simulink model "untitled"  (R2025b)
settings: Solver=VariableStepAuto  StartTime=0.0  StopTime=10.0  RelTol=1e-3
values from neighbouring files (symbols this model uses):
  K = [2.2360679775  -3.63559992725e-16  2.72862768324e-16; 1.21237084823e-16  4.08248290464  2.65354085926]    [thetad.mat]    (also in vd.mat; wd.mat; yd.mat)
  L = 0.4    [thetad.mat]    (also in vd.mat; wd.mat; yd.mat)
libraries: simulink x4, slpidlib x2
settings Model: Creator=mwali  LastModifiedBy=mwali

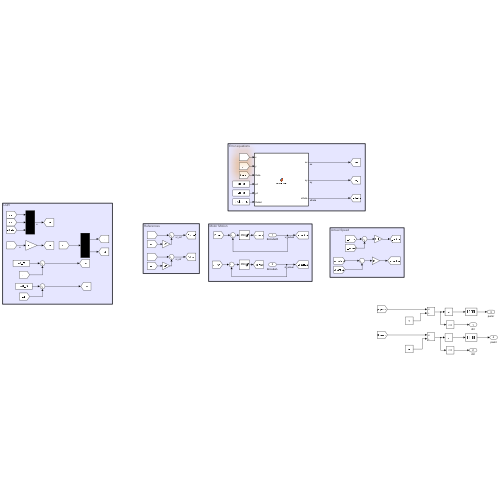
[thumbnail: Simulink's stored preview of the top-level diagram]
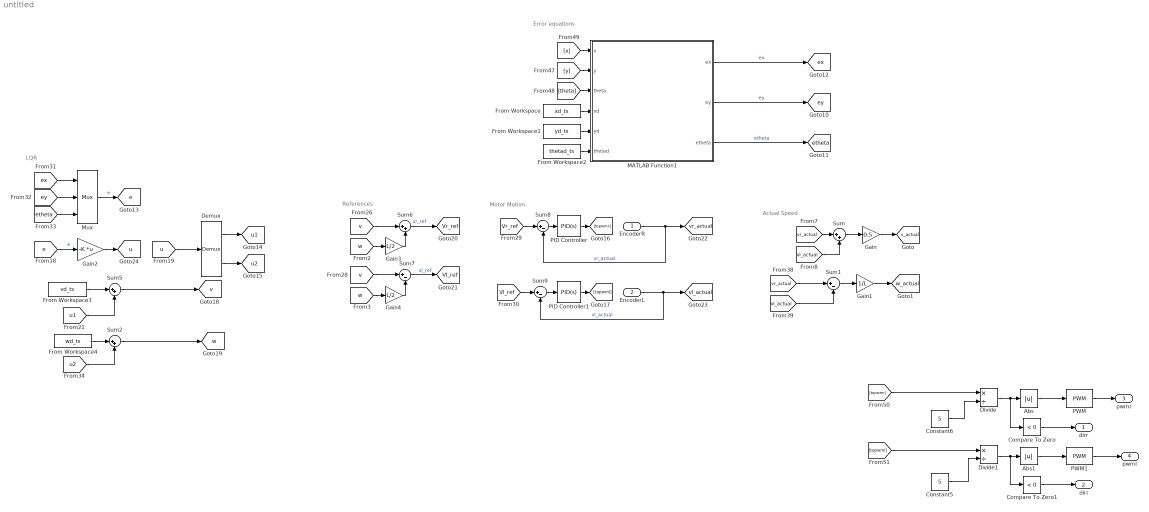
== system untitled ==
  note: LQR
  note: Actual Speed
  note: Error equations
  note: Motor Motion
  note: References
  EncoderR : Inport
  EncoderL : Inport  Port=2
  Abs : Abs  SaturateOnIntegerOverflow=off
  Abs1 : Abs  SaturateOnIntegerOverflow=off
  Compare To Zero : simulink/Logic and Bit Operations/Compare To Zero  relop=<  OutDataTypeStr=boolean
  Compare To Zero1 : simulink/Logic and Bit Operations/Compare To Zero  relop=<  OutDataTypeStr=boolean
  Constant5 : Constant  Value=5
  Constant6 : Constant  Value=5
  Demux : Demux  Outputs=2
  Divide : Product  Inputs=*/
  Divide1 : Product  Inputs=*/
  From Workspace : FromWorkspace  VariableName=xd_ts
  From Workspace1 : FromWorkspace  VariableName=yd_ts
  From Workspace2 : FromWorkspace  VariableName=thetad_ts
  From Workspace3 : FromWorkspace  VariableName=vd_ts
  From Workspace4 : FromWorkspace  VariableName=wd_ts
  Gain : Gain  Gain=0.5
  Gain1 : Gain  Gain=1/L
  Gain2 : Gain  Gain=-K  Multiplication=Matrix(K*u)
  Gain3 : Gain  Gain=L/2
  Gain4 : Gain  Gain=L/2
  MATLAB Function1 : MATLAB Function  TreatAsAtomicUnit=on
  Mux : Mux  Inputs=3
  PID Controller : slpidlib/PID Controller  Controller=PID  Form=Parallel  TimeDomain=Continuous-time  UseExternalTs=off  SampleTime=-1  IntegratorMethod=Forward Euler  FilterMethod=Forward Euler  ControllerParametersSource=internal  P=5  I=0.07  UseKiTs=off  D=0  UseExternalDerivativeSource=off  N=100  UseFilter=on  TunerSelectOption=Transfer Function Based (PID Tuner App)  InitialConditionSource=internal  InitialConditionForIntegrator=0  InitialConditionForFilter=0  DifferentiatorICPrevScaledInput=0  ExternalReset=none  TrackingMode=off  Kt=1  LimitOutput=on  SatLimitsSource=internal  UpperSaturationLimit=5  LowerSaturationLimit=-5  LinearizeAsGain=on  AntiWindupMode=clamping  Kb=1  LimitIntegrator=off  UpperIntegratorSaturationLimit=inf  LowerIntegratorSaturationLimit=-inf  POutMin=[]  POutMax=[]  IOutMin=[]  IOutMax=[]  DOutMin=[]  DOutMax=[]  NOutMin=[]  NOutMax=[]  SumOutMin=[]  SumOutMax=[]  SaturationOutMin=[]  SaturationOutMax=[]  PParamMin=[]  PParamMax=[]  IParamMin=[]  IParamMax=[]  DParamMin=[]  DParamMax=[]  NParamMin=[]  NParamMax=[]  KbParamMin=[]  KbParamMax=[]  KtParamMin=[]  KtParamMax=[]  KbOutMin=[]  KbOutMax=[]  KtOutMin=[]  KtOutMax=[]  IntegratorOutMin=[]  IntegratorOutMax=[]  FilterOutMin=[]  FilterOutMax=[]  SumI1OutMin=[]  SumI1OutMax=[]  SumI2OutMin=[]  SumI2OutMax=[]  SumI3OutMin=[]  SumI3OutMax=[]  SumI4OutMin=[]  SumI4OutMax=[]  SumDOutMin=[]  SumDOutMax=[]  DifferentiatorOutMin=[]  DifferentiatorOutMax=[]  FilterDiffOutCoefMin=[]  FilterDiffOutCoefMax=[]  ReciprocalOutMin=[]  ReciprocalOutMax=[]  SumDenOutMin=[]  SumDenOutMax=[]  SumNumOutMin=[]  SumNumOutMax=[]  DivideOutMin=[]  DivideOutMax=[]  UdiffTsProdOutMin=[]  UdiffTsProdOutMax=[]  NTsProdOutMin=[]  NTsProdOutMax=[]  UintegralTsProdOutMin=[]  UintegralTsProdOutMax=[]  UngainTsProdOutMin=[]  UngainTsProdOutMax=[]  ClampingZeroOutDataTypeStr=Inherit: Inherit via back propagation  ClampingZeroOutMin=[]  ClampingZeroOutMax=[]  FilterDenConstantOutDataTypeStr=Inherit: Inherit via back propagation  FilterDenConstantOutMin=[]  FilterDenConstantOutMax=[]  PCopyOutDataTypeStr=Inherit: Inherit via back propagation  PCopyOutMin=[]  PCopyOutMax=[]  NCopyOutDataTypeStr=Inherit: Inherit via back propagation  NCopyOutMin=[]  NCopyOutMax=[]  IntegratorContinuousStateAttributes=''  IntegratorStateMustResolveToSignalObject=off  IntegratorRTWStateStorageClass=Auto  FilterContinuousStateAttributes=''  FilterStateMustResolveToSignalObject=off  FilterRTWStateStorageClass=Auto  ParallelPVariant=InternalParameters  IdealPVariant=Disabled  IVariant=InternalParameters  DVariant=InternalParameters  IntegratorVariant=Continuous  SatVariant=Enabled  AWVariant=ContClampingParallel  PCopyVariant=Disabled  TRVariant=Disabled  FdbkBlocksVariant=Forward  IdealPFdbkVariant=Disabled  SatFdbkVariant=Disabled  DerivativeFilterVariant=ContFilter  NVariant=InternalParameters  NCopyVariant=Disabled  FilterICVariant=InternalICsFilter  IntegratorICVariant=InternalICs  ExternalResetVariant=Disabled  TRSumVariant=Passthrough  SumFdbkVariant=Disabled  SumVariant=Sum_PID  TsampFilterVariant=InternalTs  TsampNgainVariant=Passthrough  TsampIntegralVariant=Disabled_SignalSpec  ExternalSaturationOutDataTypeStr=Inherit: Same as second input  DerivativeSourceVariant=ErrorSignal  PreIntVariant=InternalPreInt
  PID Controller1 : slpidlib/PID Controller  Controller=PID  Form=Parallel  TimeDomain=Continuous-time  UseExternalTs=off  SampleTime=-1  IntegratorMethod=Forward Euler  FilterMethod=Forward Euler  ControllerParametersSource=internal  P=5  I=0.07  UseKiTs=off  D=0  UseExternalDerivativeSource=off  N=100  UseFilter=on  TunerSelectOption=Transfer Function Based (PID Tuner App)  InitialConditionSource=internal  InitialConditionForIntegrator=0  InitialConditionForFilter=0  DifferentiatorICPrevScaledInput=0  ExternalReset=none  TrackingMode=off  Kt=1  LimitOutput=on  SatLimitsSource=internal  UpperSaturationLimit=5  LowerSaturationLimit=-5  LinearizeAsGain=on  AntiWindupMode=clamping  Kb=1  LimitIntegrator=off  UpperIntegratorSaturationLimit=inf  LowerIntegratorSaturationLimit=-inf  POutMin=[]  POutMax=[]  IOutMin=[]  IOutMax=[]  DOutMin=[]  DOutMax=[]  NOutMin=[]  NOutMax=[]  SumOutMin=[]  SumOutMax=[]  SaturationOutMin=[]  SaturationOutMax=[]  PParamMin=[]  PParamMax=[]  IParamMin=[]  IParamMax=[]  DParamMin=[]  DParamMax=[]  NParamMin=[]  NParamMax=[]  KbParamMin=[]  KbParamMax=[]  KtParamMin=[]  KtParamMax=[]  KbOutMin=[]  KbOutMax=[]  KtOutMin=[]  KtOutMax=[]  IntegratorOutMin=[]  IntegratorOutMax=[]  FilterOutMin=[]  FilterOutMax=[]  SumI1OutMin=[]  SumI1OutMax=[]  SumI2OutMin=[]  SumI2OutMax=[]  SumI3OutMin=[]  SumI3OutMax=[]  SumI4OutMin=[]  SumI4OutMax=[]  SumDOutMin=[]  SumDOutMax=[]  DifferentiatorOutMin=[]  DifferentiatorOutMax=[]  FilterDiffOutCoefMin=[]  FilterDiffOutCoefMax=[]  ReciprocalOutMin=[]  ReciprocalOutMax=[]  SumDenOutMin=[]  SumDenOutMax=[]  SumNumOutMin=[]  SumNumOutMax=[]  DivideOutMin=[]  DivideOutMax=[]  UdiffTsProdOutMin=[]  UdiffTsProdOutMax=[]  NTsProdOutMin=[]  NTsProdOutMax=[]  UintegralTsProdOutMin=[]  UintegralTsProdOutMax=[]  UngainTsProdOutMin=[]  UngainTsProdOutMax=[]  ClampingZeroOutDataTypeStr=Inherit: Inherit via back propagation  ClampingZeroOutMin=[]  ClampingZeroOutMax=[]  FilterDenConstantOutDataTypeStr=Inherit: Inherit via back propagation  FilterDenConstantOutMin=[]  FilterDenConstantOutMax=[]  PCopyOutDataTypeStr=Inherit: Inherit via back propagation  PCopyOutMin=[]  PCopyOutMax=[]  NCopyOutDataTypeStr=Inherit: Inherit via back propagation  NCopyOutMin=[]  NCopyOutMax=[]  IntegratorContinuousStateAttributes=''  IntegratorStateMustResolveToSignalObject=off  IntegratorRTWStateStorageClass=Auto  FilterContinuousStateAttributes=''  FilterStateMustResolveToSignalObject=off  FilterRTWStateStorageClass=Auto  ParallelPVariant=InternalParameters  IdealPVariant=Disabled  IVariant=InternalParameters  DVariant=InternalParameters  IntegratorVariant=Continuous  SatVariant=Enabled  AWVariant=ContClampingParallel  PCopyVariant=Disabled  TRVariant=Disabled  FdbkBlocksVariant=Forward  IdealPFdbkVariant=Disabled  SatFdbkVariant=Disabled  DerivativeFilterVariant=ContFilter  NVariant=InternalParameters  NCopyVariant=Disabled  FilterICVariant=InternalICsFilter  IntegratorICVariant=InternalICs  ExternalResetVariant=Disabled  TRSumVariant=Passthrough  SumFdbkVariant=Disabled  SumVariant=Sum_PID  TsampFilterVariant=InternalTs  TsampNgainVariant=Passthrough  TsampIntegralVariant=Disabled_SignalSpec  ExternalSaturationOutDataTypeStr=Inherit: Same as second input  DerivativeSourceVariant=ErrorSignal  PreIntVariant=InternalPreInt
  PWM : simulink/Discontinuities/PWM  DisableCoverage=on  Period=1/500  InitialDelay=0  DisallowZeroDutyCycle=off  RunAtFixedTimeIntervals=on  SampleTime=0.1
  PWM1 : simulink/Discontinuities/PWM  DisableCoverage=on  Period=1/500  InitialDelay=0  DisallowZeroDutyCycle=off  RunAtFixedTimeIntervals=on  SampleTime=0.1
  Sum{,2,5..6} (4 alike) : Sum  Inputs=|++
  Sum{1,7..9} (4 alike) : Sum  Inputs=|+-
  dirr : Outport
  dirl : Outport  Port=2
  pwmr : Outport  Port=3
  pwml : Outport  Port=4
  tag scope: Vl_ref=global, Vr_ref=global, e=global, etheta=global, ex=global, ey=global, u1=global, u2=global, u=global, v=global, v_actual=global, vl_actual=global, vr_actual=global, w=global, w_actual=global
  wires:
  [u1] -> Sum5/2
  From Workspace1/1 -> MATLAB Function1/5(yd)
  [Vr_ref] -> Sum8/1
  Sum5/1 -> [v]
  Abs1/1 -> PWM1/1
  EncoderL/1 -> [vl_actual], Sum9/2  "vl_actual"
  Sum9/1 -> PID Controller1/1
  [theta] -> MATLAB Function1/3(theta)
  [Vl_ref] -> Sum9/1
  [e] -> Gain2/1  "e"
  Demux/1 -> [u1]
  [vl_actual] -> Sum/2
  [u2] -> Sum2/2
  Mux/1 -> [e]  "e"
  [vr_actual] -> Sum/1
  From Workspace3/1 -> Sum5/1
  [x] -> MATLAB Function1/1(x)
  [etheta] -> Mux/3
  Compare To Zero/1 -> dirr/1
  Constant5/1 -> Divide1/2
  MATLAB Function1/2(ey) -> [ey]  "ey"
  EncoderR/1 -> [vr_actual], Sum8/2  "vr_actual"
  PID Controller1/1 -> [topwml]
  [u] -> Demux/1
  [v] -> Sum6/1
  Gain/1 -> [v_actual]
  Abs/1 -> PWM/1
  From Workspace/1 -> MATLAB Function1/4(xd)
  From Workspace4/1 -> Sum2/1
  Sum7/1 -> [Vl_ref]  "vl_ref"
  [vl_actual] -> Sum1/2
  [topwml] -> Divide1/1
  [w] -> Gain3/1
  Gain2/1 -> [u]
  Gain3/1 -> Sum6/2
  Divide1/1 -> Abs1/1, Compare To Zero1/1
  [vr_actual] -> Sum1/1
  [y] -> MATLAB Function1/2(y)
  Sum8/1 -> PID Controller/1
  [ex] -> Mux/1
  Demux/2 -> [u2]
  Compare To Zero1/1 -> dirl/1
  Sum1/1 -> Gain1/1
  MATLAB Function1/3(etheta) -> [etheta]  "etheta"
  Sum6/1 -> [Vr_ref]  "vr_ref"
  Sum2/1 -> [w]
  [ey] -> Mux/2
  Constant6/1 -> Divide/2
  Gain4/1 -> Sum7/2
  [topwmr] -> Divide/1
  PWM/1 -> pwmr/1
  PWM1/1 -> pwml/1
  [v] -> Sum7/1
  From Workspace2/1 -> MATLAB Function1/6(thetad)
  [w] -> Gain4/1
  Divide/1 -> Abs/1, Compare To Zero/1
  MATLAB Function1/1(ex) -> [ex]  "ex"
  PID Controller/1 -> [topwmr]
  Sum/1 -> Gain/1
  Gain1/1 -> [w_actual]

== matlab function untitled/MATLAB Function1 ==
  data: x input; ex output; y input; theta input; xd input; yd input; thetad input; ey output; etheta output
function [ex, ey, etheta] = calcError(x, y, theta, xd, yd, thetad)

dx = x - xd;
dy = y - yd;

ex =  cos(thetad)*dx + sin(thetad)*dy;
ey = -sin(thetad)*dx + cos(thetad)*dy;

etheta = atan2(sin(theta - thetad), cos(theta - thetad));
